simulink model "ORFS_Model"  (R2023b)
settings: Solver=FixedStepAuto  StartTime=0.0  StopTime=t_Total  FixedStep=dt  RelTol=1e-3
undefined symbols (not defined in the file): Drone, dt, Flapping, g, rho, Tail, u_0, Wing, X_0
libraries: simulink_extras x12, spsMeanLib x10, spsMeanVariableFrequencyLib x8, matrix_library x1, aerolibanimutils x1
settings Model: PacingRate=10  Creator=iwl  LastModifiedBy=iwl
settings DataIOCC: SaveState=on
settings ModelReferenceCC: EnableRefExpFcnMdlSchedulingChecks=on

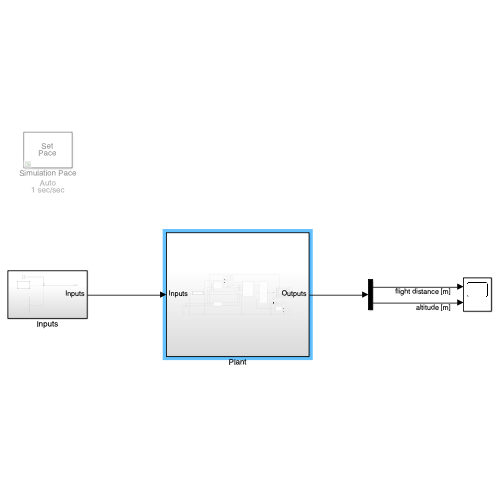
[thumbnail: Simulink's stored preview of the top-level diagram]
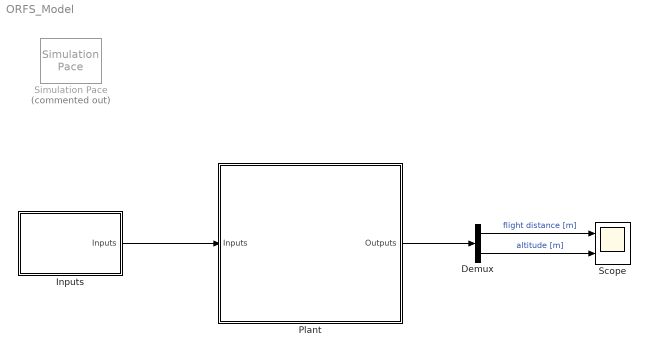
== system ORFS_Model ==
  Demux : Demux  Outputs=2
  Inputs : Subsystem
  Plant : Subsystem
  Scope : Scope  NumInputPorts=2
  Simulation Pace : aerolibanimutils/Simulation Pace  Commented=on  SimulationPace=1  SleepMode=Auto  OutputPaceError=off  SampleTime=dt
  wires:
  Plant/1(Outputs) -> Demux/1
  Demux/1 -> Scope/1  "flight distance [m]"
  Inputs/1(Inputs) -> Plant/1(Inputs)
  Demux/2 -> Scope/2  "altitude [m]"

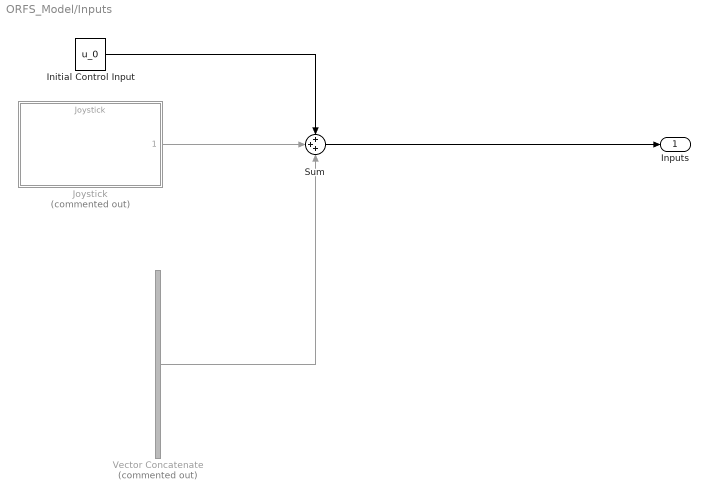
== system ORFS_Model/Inputs ==
  Initial Control Input : Constant  Value=u_0
  Joystick : ModelReference  Commented=on  ModelNameDialog=Joystick.slx  SimulationMode=Normal  ModelReferenceVersion=4.1
  Sum : Sum  Inputs=+++
  Vector Concatenate : Concatenate  Commented=on  NumInputs=3
  Inputs : Outport
  wires:
  Sum/1 -> Inputs/1
  Initial Control Input/1 -> Sum/1
  Vector Concatenate/1 -> Sum/3
  Joystick/1 -> Sum/2

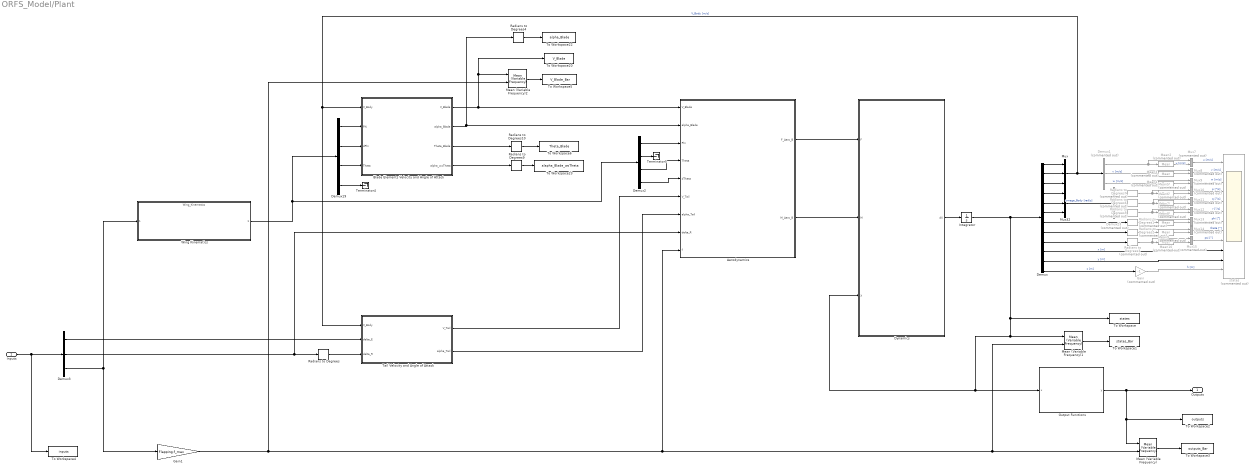
== system ORFS_Model/Plant ==
  Inputs : Inport
  Aerodynamics : Subsystem
  Blade Elements Velocity and Angle of Attack : MATLAB Function  TreatAsAtomicUnit=on
  Demux : Demux  Outputs=12
  Demux1 : Demux  Commented=on  Outputs=3
  Demux19 : Demux
  Demux2 : Demux
  Demux23 : Demux  Commented=on  Outputs=3
  Demux3 : Demux  Outputs=3
  Dynamics : MATLAB Function  TreatAsAtomicUnit=on
  Gain : Gain  Commented=on  Gain=-1
  Gain1 : Gain  Gain=Flapping.f_max
  Integrator : Integrator  InitialCondition=X_0
  Mean (Variable Frequency) : spsMeanVariableFrequencyLib/Mean (Variable Frequency)  Finit=Flapping.f_max* u_0(3)  Fmin=0.01  Vinit=0  Ts=0.01
      settings: LibrarySourceBlock=|
      | sps_lib/Sensors and Measurements/Mean
      | (Variable Frequency)
  Mean (Variable Frequency)1 : spsMeanVariableFrequencyLib/Mean (Variable Frequency)  Finit=Flapping.f_max* u_0(3)  Fmin=0.01  Vinit=0  Ts=0.01
      settings: LibrarySourceBlock=|
      | sps_lib/Sensors and Measurements/Mean
      | (Variable Frequency)
  Mean (Variable Frequency)2 : spsMeanVariableFrequencyLib/Mean (Variable Frequency)  Finit=Flapping.f_max* u_0(3)  Fmin=0.01  Vinit=0  Ts=0.01
      settings: LibrarySourceBlock=|
      | sps_lib/Sensors and Measurements/Mean
      | (Variable Frequency)
  Mean{2..10} (9 alike) : spsMeanLib/Mean  Commented=on  Freq=f_max  Vinit=0  Ts=0
  Mux : Mux  Inputs=3
  Mux{7..15} (9 alike) : Mux  Commented=on  Inputs=2
  Mux32 : Mux  Inputs=3
  Output Functions : MATLAB Function  TreatAsAtomicUnit=on
  Radians to Degrees{,4,9..10} (4 alike) : simulink_extras/Transformations/Radians to Degrees
  Radians to Degrees{1..3,5..7} (6 alike) : simulink_extras/Transformations/Radians to Degrees  Commented=on
  Tail Velocity and Angle of Attack : MATLAB Function  TreatAsAtomicUnit=on
  Terminator4 : Terminator
  Terminator5 : Terminator
  To Workspace : ToWorkspace  VariableName=states  SampleTime=-1
  To Workspace1 : ToWorkspace  VariableName=states_Bar  SampleTime=-1
  To Workspace2 : ToWorkspace  VariableName=outputs  SampleTime=-1
  To Workspace20 : ToWorkspace  VariableName=V_Blade  SampleTime=-1
  To Workspace22 : ToWorkspace  VariableName=alpha_Blade  SampleTime=-1
  To Workspace23 : ToWorkspace  VariableName=alapha_Blade_woTheta  SampleTime=-1
  To Workspace3 : ToWorkspace  VariableName=outputs_Bar  SampleTime=-1
  To Workspace4 : ToWorkspace  VariableName=inputs  SampleTime=-1
  To Workspace5 : ToWorkspace  VariableName=V_Blade_Bar  SampleTime=-1
  To Workspace6 : ToWorkspace  VariableName=Theta_Blade  SampleTime=-1
  Wing Kinematics : ModelReference  ModelNameDialog=Wing_Kinematics.slx  SimulationMode=Normal  ModelReferenceVersion=4.6
  states : Scope  Commented=on  NumInputPorts=12
  Outputs : Outport
  wires:
  Mean (Variable Frequency)1/1 -> To Workspace1/1
  Demux19/3 -> Blade Elements Velocity and Angle of Attack/4(Theta)
  Demux19/2 -> Blade Elements Velocity and Angle of Attack/3(dPhi)
  Demux23/2 -> Radians to Degrees6/1
  Demux/5 -> Mux32/2
  Mux7/1 -> states/1  "u [m/s]"
  Mean4/1 -> Mux9/2
  Demux/9 -> Radians to Degrees3/1
  Demux2/2 -> Terminator5/1
  Demux1/1 -> Mean2/1, Mux7/1  "u [m/s]"
  Mean9/1 -> Mux14/2
  Aerodynamics/2(M_Aero_B) -> Dynamics/2(M)
  Demux/3 -> Mux/3
  Mean2/1 -> Mux7/2
  Demux/6 -> Mux32/3
  Radians to Degrees4/1 -> To Workspace22/1
  Demux/7 -> Radians to Degrees1/1
  Mux14/1 -> states/8  "theta [°]"
  Demux2/1 -> Aerodynamics/3(Phi)
  Demux19/4 -> Terminator4/1
  Mean3/1 -> Mux8/2
  Mean5/1 -> Mux10/2
  Mean10/1 -> Mux15/2
  Blade Elements Velocity and Angle of Attack/4(alpha_woTheta) -> Radians to Degrees9/1
  Mux11/1 -> states/5  "q [°/s]"
  Radians to Degrees5/1 -> Mux12/1, Mean7/1
  Demux2/4 -> Aerodynamics/5(dTheta)
  Radians to Degrees1/1 -> Mux13/1, Mean8/1
  Radians to Degrees6/1 -> Mux11/1, Mean6/1
  Dynamics/1(dX) -> Integrator/1
  Integrator/1 -> Dynamics/3(X), Output Functions/1(x), Mean (Variable Frequency)1/2, To Workspace/1, Demux/1
  Demux1/2 -> Mean3/1, Mux8/1  "v [m/s]"
  Mux12/1 -> states/6  "r [°/s]"
  Mux10/1 -> states/4  "p [°/s]"
  Mux9/1 -> states/3  "w [m/s]"
  Radians to Degrees2/1 -> Mux14/1, Mean9/1
  Demux1/3 -> Mean4/1, Mux9/1  "w [m/s]"
  Mean7/1 -> Mux12/2
  Demux/12 -> Gain/1  "z [m]"
  Demux/4 -> Mux32/1
  Demux/2 -> Mux/2
  Wing Kinematics/1 -> Demux2/1, Demux19/1
  Demux19/1 -> Blade Elements Velocity and Angle of Attack/2(Phi)
  Mux15/1 -> states/9  "psi [°]"
  Demux2/3 -> Aerodynamics/4(Theta)
  Demux/10 -> states/10  "x [m]"
  Mean8/1 -> Mux13/2
  Mux32/1 -> Demux23/1  "omega_Body [rad/s]"
  Blade Elements Velocity and Angle of Attack/3(Theta_Blade) -> Radians to Degrees10/1
  Mux/1 -> Demux1/1, Blade Elements Velocity and Angle of Attack/1(V_Body), Tail Velocity and Angle of Attack/1(V_Body)  "V_Body [m/s]"
  Demux23/1 -> Radians to Degrees7/1
  Demux/1 -> Mux/1
  Blade Elements Velocity and Angle of Attack/2(alpha_Blade) -> Radians to Degrees4/1, Aerodynamics/2(alpha_Blade)
  Aerodynamics/1(F_Aero_B) -> Dynamics/1(F)
  Mean6/1 -> Mux11/2
  Radians to Degrees7/1 -> Mux10/1, Mean5/1
  Mux8/1 -> states/2  "v [m/s]"
  Mux13/1 -> states/7  "phi [°]"
  Demux/8 -> Radians to Degrees2/1
  Radians to Degrees3/1 -> Mux15/1, Mean10/1
  Demux23/3 -> Radians to Degrees5/1
  Output Functions/1(y) -> Outputs/1, Mean (Variable Frequency)/2, To Workspace2/1
  Gain/1 -> states/12  "h [m]"
  Radians to Degrees/1 -> Tail Velocity and Angle of Attack/3(delta_R)
  Tail Velocity and Angle of Attack/1(V_Tail) -> Aerodynamics/6(V_Tail)
  Tail Velocity and Angle of Attack/2(alpha_Tail) -> Aerodynamics/7(alpha_Tail)
  Inputs/1 -> To Workspace4/1, Demux3/1
  Demux3/1 -> Tail Velocity and Angle of Attack/2(delta_E)
  Demux3/2 -> Radians to Degrees/1, Aerodynamics/8(delta_R)
  Radians to Degrees9/1 -> To Workspace23/1
  Radians to Degrees10/1 -> To Workspace6/1
  Mean (Variable Frequency)/1 -> To Workspace3/1
  Demux3/3 -> Gain1/1, Wing Kinematics/1
  Blade Elements Velocity and Angle of Attack/1(V_Blade) -> Aerodynamics/1(V_Blade), To Workspace20/1, Mean (Variable Frequency)2/2
  Gain1/1 -> Mean (Variable Frequency)2/1, Aerodynamics/9(f), Mean (Variable Frequency)1/1, Mean (Variable Frequency)/1
  Mean (Variable Frequency)2/1 -> To Workspace5/1
  Demux/11 -> states/11  "y [m]"

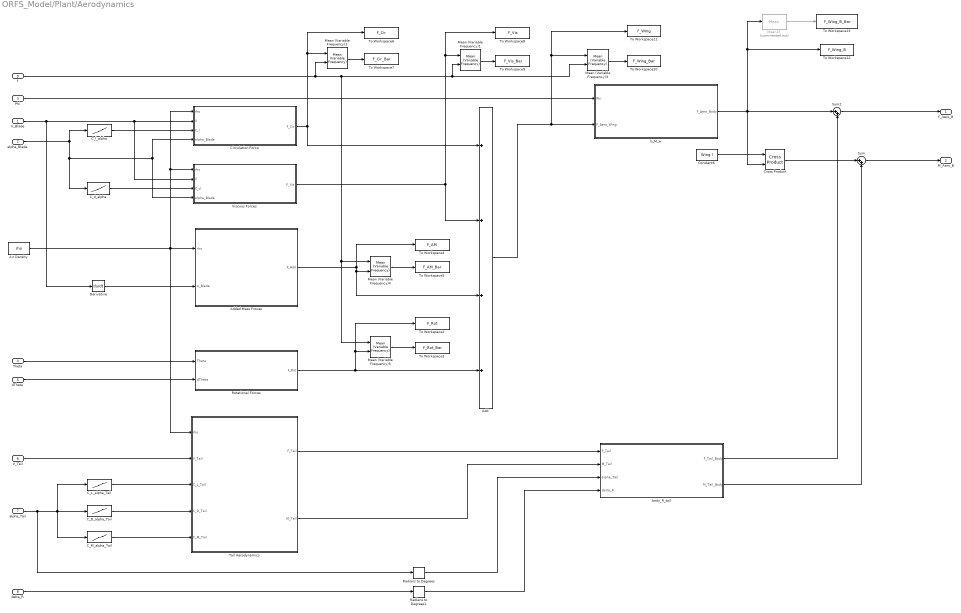
== system ORFS_Model/Plant/Aerodynamics ==
  V_Blade : Inport
  alpha_Blade : Inport  Port=2
  Phi : Inport  Port=3
  Theta : Inport  Port=4
  dTheta : Inport  Port=5
  V_Tail : Inport  Port=6
  alpha_Tail : Inport  Port=7
  delta_R : Inport  Port=8
  f : Inport  Port=9
  Add : Sum  Inputs=++++
  Added Mass Froces : MATLAB Function  TreatAsAtomicUnit=on
  Air Density : Constant  Value=rho
  C_D_alpha_Tail : Lookup_n-D  NumberOfTableDimensions=1  BreakpointsForDimension1=Tail.alpha  Table=Tail.C_D  InternalRulePriority=Speed  RndMeth=Simplest
  C_L_alpha_Tail : Lookup_n-D  NumberOfTableDimensions=1  BreakpointsForDimension1=Tail.alpha  Table=Tail.C_L  InternalRulePriority=Speed  RndMeth=Simplest
  C_M_alpha_Tail : Lookup_n-D  NumberOfTableDimensions=1  BreakpointsForDimension1=Tail.alpha  Table=Tail.C_M  InternalRulePriority=Speed  RndMeth=Simplest
  C_d_alpha : Lookup_n-D  NumberOfTableDimensions=1  BreakpointsForDimension1=Wing.alpha_C_d  Table=Wing.C_d  InternalRulePriority=Speed  RndMeth=Simplest
  C_l_alpha : Lookup_n-D  NumberOfTableDimensions=1  BreakpointsForDimension1=Wing.alpha_C_l  Table=Wing.C_l  InternalRulePriority=Speed  RndMeth=Simplest
  Circulation Force : MATLAB Function  TreatAsAtomicUnit=on
  Constant6 : Constant  Value=Wing.l
  Cross Product : matrix_library/Cross Product
  Derivative : Derivative
  Mean (Variable Frequency){1..5} (5 alike) : spsMeanVariableFrequencyLib/Mean (Variable Frequency)  Finit=Flapping.f_max* u_0(3)  Fmin=0.01  Vinit=0  Ts=0.01
      settings: LibrarySourceBlock=|
      | sps_lib/Sensors and Measurements/Mean
      | (Variable Frequency)
  Mean15 : spsMeanLib/Mean  Commented=on  Freq=f_max  Vinit=0  Ts=0
  Radians to Degrees : simulink_extras/Transformations/Radians to Degrees
  Radians to Degrees1 : simulink_extras/Transformations/Radians to Degrees
  Rotational Forces : MATLAB Function  TreatAsAtomicUnit=on
  Sum : Sum  Inputs=|++
  Sum2 : Sum  Inputs=|++
  Tail Aerodynamics : MATLAB Function  TreatAsAtomicUnit=on
  To Workspace10 : ToWorkspace  VariableName=F_Wing_Bar  SampleTime=-1
  To Workspace11 : ToWorkspace  VariableName=F_WIng  SampleTime=-1
  To Workspace12 : ToWorkspace  VariableName=F_Wing_B  SampleTime=-1
  To Workspace13 : ToWorkspace  VariableName=F_Wing_B_Bar  SampleTime=-1
  To Workspace2 : ToWorkspace  VariableName=F_Rot  SampleTime=-1
  To Workspace3 : ToWorkspace  VariableName=F_Rot_Bar  SampleTime=-1
  To Workspace4 : ToWorkspace  VariableName=F_AM  SampleTime=-1
  To Workspace5 : ToWorkspace  VariableName=F_AM_Bar  SampleTime=-1
  To Workspace6 : ToWorkspace  VariableName=F_Cir  SampleTime=-1
  To Workspace7 : ToWorkspace  VariableName=F_Cir_Bar  SampleTime=-1
  To Workspace8 : ToWorkspace  VariableName=F_Vis  SampleTime=-1
  To Workspace9 : ToWorkspace  VariableName=F_Vis_Bar  SampleTime=-1
  Viscous Forces : MATLAB Function  TreatAsAtomicUnit=on
  b_M_w : MATLAB Function  TreatAsAtomicUnit=on
  body_R_tail : MATLAB Function  TreatAsAtomicUnit=on
  F_Aero_B : Outport
  M_Aero_B : Outport  Port=2
  wires:
  V_Tail/1 -> Tail Aerodynamics/2(V_Tail)
  Theta/1 -> Rotational Forces/1(Theta)
  C_L_alpha_Tail/1 -> Tail Aerodynamics/3(C_L_Tail)
  C_M_alpha_Tail/1 -> Tail Aerodynamics/5(C_M_Tail)
  Mean15/1 -> To Workspace13/1
  Phi/1 -> b_M_w/1(Phi)
  Tail Aerodynamics/1(F_Tail) -> body_R_tail/1(F_Tail)
  Constant6/1 -> Cross Product/1
  V_Blade/1 -> Circulation Force/2(V), Viscous Forces/2(V), Derivative/1
  Mean (Variable Frequency)2/1 -> To Workspace7/1
  Mean (Variable Frequency)4/1 -> To Workspace5/1
  C_d_alpha/1 -> Viscous Forces/3(C_d)
  Viscous Forces/1(F_Vis) -> Add/2, To Workspace8/1, Mean (Variable Frequency)1/2
  Mean (Variable Frequency)5/1 -> To Workspace3/1
  Rotational Forces/1(F_Rot) -> To Workspace2/1, Mean (Variable Frequency)5/2, Add/4
  alpha_Tail/1 -> Radians to Degrees/1, C_L_alpha_Tail/1, C_D_alpha_Tail/1, C_M_alpha_Tail/1
  delta_R/1 -> Radians to Degrees1/1
  Air Density/1 -> Circulation Force/1(rho), Viscous Forces/1(rho), Tail Aerodynamics/1(rho), Added Mass Froces/1(rho)
  Mean (Variable Frequency)3/1 -> To Workspace10/1
  C_D_alpha_Tail/1 -> Tail Aerodynamics/4(C_D_Tail)
  Circulation Force/1(F_Cir) -> To Workspace6/1, Mean (Variable Frequency)2/2, Add/1
  C_l_alpha/1 -> Circulation Force/3(C_l)
  alpha_Blade/1 -> C_l_alpha/1, C_d_alpha/1, Viscous Forces/4(alpha_Blade), Circulation Force/4(alpha_Blade)
  Derivative/1 -> Added Mass Froces/2(a_Blade)
  Mean (Variable Frequency)1/1 -> To Workspace9/1
  Added Mass Froces/1(F_Add) -> Mean (Variable Frequency)4/2, Add/3, To Workspace4/1
  dTheta/1 -> Rotational Forces/2(dTheta)
  Sum2/1 -> F_Aero_B/1
  body_R_tail/1(F_Tail_Body) -> Sum2/2
  Radians to Degrees/1 -> body_R_tail/3(alpha_Tail)
  Radians to Degrees1/1 -> body_R_tail/4(delta_R)
  body_R_tail/2(M_Tail_Body) -> Sum/2
  Add/1 -> b_M_w/2(F_Aero_Wing), Mean (Variable Frequency)3/2, To Workspace11/1
  Cross Product/1 -> Sum/1
  Tail Aerodynamics/2(M_Tail) -> body_R_tail/2(M_Tail)
  Sum/1 -> M_Aero_B/1
  b_M_w/1(F_Aero_Body) -> Cross Product/2, Sum2/1, Mean15/1, To Workspace12/1
  f/1 -> Mean (Variable Frequency)3/1, Mean (Variable Frequency)1/1, Mean (Variable Frequency)4/1, Mean (Variable Frequency)5/1, Mean (Variable Frequency)2/1

== matlab function ORFS_Model/Plant/Aerodynamics/Tail Aerodynamics ==
  data: rho input; F_Tail output; V_Tail input; C_L_Tail input; C_D_Tail input; C_M_Tail input; M_Tail output; Tail parameter
function [F_Tail, M_Tail] = Aerodynamic_Tail(rho, V_Tail, C_L_Tail, C_D_Tail, C_M_Tail, Tail)
    

    C_L = C_L_Tail;
    C_Y = 0;
    C_D = C_D_Tail;

    C_ML = 0;
    C_MM = C_M_Tail;
    C_MN = 0;
    
    F_Tail = 0.5* rho* norm(V_Tail)^2* Tail.S* [-C_D; C_Y; -C_L];

    M_Tail = 0.5* rho* norm(V_Tail)^2* Tail.S* Tail.b * [C_ML; C_MM; C_MN] + cross(Tail.l, F_Tail);

end

== matlab function ORFS_Model/Plant/Aerodynamics/Viscous Forces ==
  data: rho input; F_Vis output; V input; C_d input; alpha_Blade input; Wing parameter
function F_Vis   = Viscous(rho, V, C_d, alpha_Blade, Wing)
       
    dF_Vis = sum(0.5 * rho * V .* V .* C_d .* Wing.c * Wing.dr) .* [-cos(alpha_Blade); zeros(1, size(alpha_Blade, 2)); -sin(alpha_Blade)];

    F_Vis = 2* sum(dF_Vis, 2);
    
end

== matlab function ORFS_Model/Plant/Aerodynamics/body_R_tail ==
  data: F_Tail input; M_Tail input; alpha_Tail input; delta_R input; F_Tail_Body output; M_Tail_Body output
function [F_Tail_Body, M_Tail_Body]   = Transformation_Tail_to_Body(F_Tail, M_Tail, alpha_Tail, delta_R)
    
    F_Tail_Body = rotx(delta_R)* roty(alpha_Tail)* F_Tail;

    M_Tail_Body = rotx(delta_R)* roty(alpha_Tail)* M_Tail;
    %M_Tail_Body = rotx(-delta_R)* M_Tail;

end

== matlab function ORFS_Model/Plant/Dynamics ==
  data: F input; dX output; M input; X input; Drone parameter; g parameter
function dX  = Dynamics(F, M, X, Drone, g)

    % X = [u; v; w; p; q; r; Phi; Theta; Psi; x; y; z]

    u = X(1);
    v = X(2);
    w = X(3);
    p = X(4);
    q = X(5);
    r = X(6);
    phi = X(7);
    theta = X(8);
    psi = X(9);

    dX = zeros(12, 1);

%     M_BE = [1, 0, 0;
%             0, cos(phi), sin(phi);
%             0, -sin(phi), cos(phi)]* ...
%            [cos(theta), 0, -sin(theta);
%             0, 1, 0;
%             sin(theta), 0, cos(theta)]* ...
%            [cos(psi), sin(psi), 0;
%             -sin(psi), cos(psi),0;
%             0,0,1];
    M_EB = [cos(psi)* cos(theta), cos(psi)* sin(theta)* sin(phi) - sin(psi)* cos(phi), cos(psi)* sin(theta)* cos(phi) + sin(psi)* sin(phi);
            sin(psi)* cos(theta), sin(psi)* sin(theta)* sin(phi) + cos(psi)* cos(phi), sin(psi)* sin(theta)* cos(phi) - cos(psi)* sin(phi);
                     -sin(theta),                                 cos(theta)*sin(phi),                                cos(theta)* cos(phi)];
    
    % translational dynamics
    dX(1:3) = F / Drone.m + g * [-sin(theta); sin(phi)* cos(theta); cos(phi)* cos(theta)] - cross([p; q; r], [u; v; w]);

    % rotational dynamics
    dX(4:6) = Drone.I \ (M - cross([p; q; r], (Drone.I* [p; q; r])));
    
    % rotational kinematics
    dX(7:9) = [1, sin(phi)* tan(theta), cos(phi)* tan(theta);
               0,             cos(phi),            -sin(phi);
               0, sin(phi)/ cos(theta), cos(phi)/ cos(theta)]* [p; q; r];

    % translational kinematics
    % dX(10:12) = M_BE \ [u; v; w];
    dX(10:12) = M_EB * [u; v; w];

end

== matlab function ORFS_Model/Plant/Output Functions ==
  data: x input; y output
function y = Output_Function(x)

    num_Outputs = 2;

    y = zeros(num_Outputs, 1);

    y(1) = x(10);
    y(2) = -x(12);

end

== matlab function ORFS_Model/Plant/Tail Velocity and Angle of Attack ==
  data: V_Body input; delta_E input; V_Tail output; alpha_Tail output; delta_R input; Tail parameter
function [V_Tail, alpha_Tail]  = V_alpha_Tail(V_Body, delta_E, delta_R, Tail)
    
    V_Tail = rotx(-delta_R)* V_Body;

    alpha_Tail = delta_E + Tail.alpha_mount + atan2(V_Tail(3), V_Tail(1));
    
end

== matlab function ORFS_Model/Plant/Blade Elements Velocity and Angle of Attack ==
  data: V_Body input; Phi input; dPhi input; Theta input; V_Blade output; alpha_Blade output; Theta_Blade output; alpha_woTheta output; Wing parameter
function [V_Blade, alpha_Blade, Theta_Blade, alpha_woTheta] = V_alpha_Wing(V_Body, Phi, dPhi, Theta, Wing)

    %% in local wing frame
    V_Flapping = Wing.r* dPhi .* [0; 0; 1];
    V_Body_W = [1 0 0; 0 cos(Phi) sin(Phi); 0 -sin(Phi) cos(Phi)] * V_Body;
    V_Blade = [V_Body_W(1); 0; V_Body_W(3)] + V_Flapping;

    %% in body frame
    % V_Flapping = r* dPhi .* [0; 0; cos(Phi)];
    % V_Total = [V(1); 0; V(3)] + V_Flapping;
    
    %% aoa
    Theta_Blade = Theta * Wing.r / (Wing.b / 2);

    alpha_Blade = atan2(V_Blade(3,:), V_Blade(1,:)) + Theta_Blade;
    alpha_woTheta = atan2(V_Blade(3,:), V_Blade(1,:));

end

== matlab function ORFS_Model/Plant/Aerodynamics/Circulation Force ==
  data: F_Cir output; rho input; V input; C_l input; alpha_Blade input; Wing parameter
function F_Cir = Circulation(rho, V, C_l, alpha_Blade, Wing)
    
    % forces on each blade element in WING frame
    dF_Cir = sum(0.5 * rho * V .* V .* C_l .* Wing.c * Wing.dr) .* [sin(alpha_Blade); zeros(1, size(alpha_Blade, 2)); -cos(alpha_Blade)];

    % dM_Circ = corss(l, dF_Circ);

    F_Cir = 2* sum(dF_Cir, 2);

    % M_Circ = 2 * sum(dM_Circ, 2);
    
end

== matlab function ORFS_Model/Plant/Aerodynamics/Added Mass Froces ==
  data: rho input; a_Blade input; Wing parameter; F_Add output
function F_Add  = Added_Mass(rho, a_Blade, Wing)

    m_11 = 0.25* pi* rho* Wing.thickness^2 * ones(size(Wing.c));
    m_22 = 0.25* pi* rho* Wing.c.^2;

    dF_Add = -[m_11.* a_Blade(1,:); zeros(1, Wing.num_Blade); m_22.* a_Blade(3,:)].* Wing.dr;
    F_Add = 2* sum(dF_Add, 2);
        
end

== matlab function ORFS_Model/Plant/Aerodynamics/Rotational Forces ==
  data: Theta input; F_Rot output; dTheta input; Wing parameter
function F_Rot = Rotational(Theta, dTheta, Wing)
    
    % c_R = 0.1666 - 0.374
    c_R = 0.1666;

    dF_Rot = c_R * dTheta .* Wing.c .* Wing.c * Wing.dr .* [cos(Theta); 0 ; sin(Theta)];
    
    F_Rot = 2* sum(dF_Rot, 2);

end

== matlab function ORFS_Model/Plant/Aerodynamics/b_M_w ==
  data: Phi input; F_Aero_Wing input; F_Aero_Body output
function F_Aero_Body = Transformation_Wing_to_Body(Phi, F_Aero_Wing)
    
    F_Aero_Body = [1 0 0; 0 cos(Phi) -sin(Phi); 0 sin(Phi) cos(Phi)] * F_Aero_Wing;

    F_Aero_Body(2) = 0;
    
end
